simulink model "motorul_de_curent"  (R2024b)
settings: Solver=VariableStepAuto  StartTime=0.0  StopTime=50  RelTol=1e-3
values from neighbouring files (symbols this model uses):
  A = [-1/Tp 1/Tp ; kp/(kc*Tc) -((1+kp/kc)/Tc)]    [pardoseala.m]    (also in simulare.m = [-1/Ta -ke/La ; km/J 0]; tema1.m = [ k1*Ti*(kE2)/(2*Ti+1) 0 ; 0 k1*Ti*(kE1)/(2*Ti+1)])
  B = [ kE/(kp * Tp) 0 ; 0 1/Tc]    [pardoseala.m]    (also in simulare.m = [kE/La 0 ; 0 -1/J]; tema1.m = [ kC/Tc 0 ; 0 -Ti])
  C = [1 0 ; 0 1]    [pardoseala.m]    (also in simulare.m; tema1.m)
  D = [0 0 ; 0 0]    [pardoseala.m]    (also in simulare.m = zeros(2); tema1.m)
  J = 0.0302    [simulare.m]
  kE = 1000    [pardoseala.m]    (also in simulare.m = 42.85)
  ke = 0.56    [simulare.m]
  km = 0.55    [simulare.m]
  Ra = 5.1    [simulare.m]
  Ta = 0.1    [simulare.m]
  Tm = 0.5    [simulare.m]
settings Model: Creator=albertrosca  LastModifiedBy=albertrosca

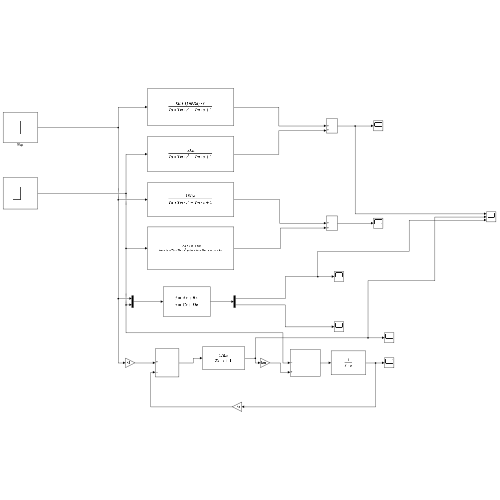
[thumbnail: Simulink's stored preview of the top-level diagram]
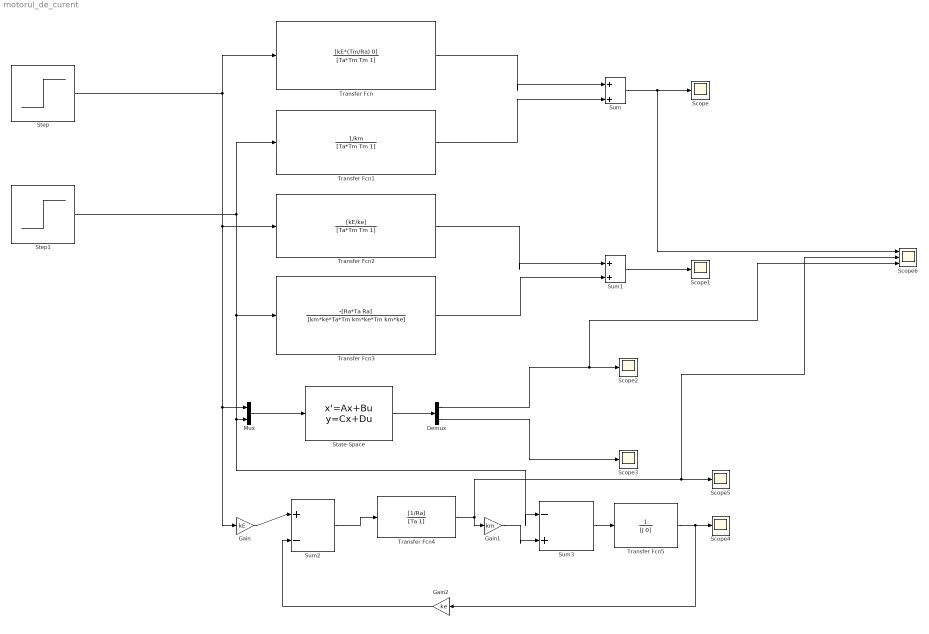
== system motorul_de_curent ==
  Demux : Demux  Outputs=2
  Gain : Gain  Gain=kE
  Gain1 : Gain  Gain=km
  Gain2 : Gain  Gain=ke
  Mux : Mux  Inputs=2
  Scope{,1..5} (6 alike) : Scope
  Scope6 : Scope  NumInputPorts=3
  State-Space : StateSpace  A=A  B=B  C=C  D=D  InitialCondition=0
  Step : Step  Time=0  After=3.5  SampleTime=0
  Step1 : Step  Time=30  SampleTime=0
  Sum : Sum  Inputs=|++
  Sum1 : Sum  Inputs=|++
  Sum2 : Sum  Inputs=|+-
  Sum3 : Sum  Inputs=|-+
  Transfer Fcn : TransferFcn  Numerator=[kE*(Tm/Ra) 0]  Denominator=[Ta*Tm Tm 1]  ContinuousStateAttributes="\"\""
  Transfer Fcn1 : TransferFcn  Numerator=1/km  Denominator=[Ta*Tm Tm 1]
  Transfer Fcn2 : TransferFcn  Numerator=[kE/ke]  Denominator=[Ta*Tm Tm 1]
  Transfer Fcn3 : TransferFcn  Numerator=-[Ra*Ta Ra]  Denominator=[km*ke*Ta*Tm km*ke*Tm km*ke]
  Transfer Fcn4 : TransferFcn  Numerator=[1/Ra]  Denominator=[Ta 1]
  Transfer Fcn5 : TransferFcn  Denominator=[J 0]
  wires:
  Step1/1 -> Sum3/1, Mux/2, Transfer Fcn3/1, Transfer Fcn1/1
  Transfer Fcn/1 -> Sum/1
  Transfer Fcn1/1 -> Sum/2
  Sum/1 -> Scope6/1, Scope/1
  Transfer Fcn2/1 -> Sum1/1
  Transfer Fcn3/1 -> Sum1/2
  Sum1/1 -> Scope1/1
  Step/1 -> Gain/1, Mux/1, Transfer Fcn2/1, Transfer Fcn/1
  Mux/1 -> State-Space/1
  State-Space/1 -> Demux/1
  Demux/1 -> Scope6/3, Scope2/1
  Demux/2 -> Scope3/1
  Transfer Fcn5/1 -> Scope4/1, Gain2/1
  Sum3/1 -> Transfer Fcn5/1
  Gain1/1 -> Sum3/2
  Transfer Fcn4/1 -> Scope6/2, Scope5/1, Gain1/1
  Sum2/1 -> Transfer Fcn4/1
  Gain/1 -> Sum2/1
  Gain2/1 -> Sum2/2
